simulink library "dspinverses"  (Simulink 8.0)
settings: Solver=ode45  SolverMode=SingleTasking  StartTime=0.0  StopTime=10.0  RelTol=1e-3
libraries: dspmtrx3 x3, dspsolvers x3
settings Model: Creator=dlinebar  LastModifiedBy=lij  ExtModeAutoUpdateStatusClock=off

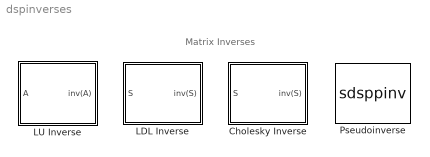
== system dspinverses ==
  note: Matrix Inverses
  " LU Inverse" : Subsystem
      mask Type: LU Inverse
      mask Description: Matrix inverse using LU factorization.
      mask Help: eval('blocksethelp');
      mask Display:
      | text(0.25,0.85,'General')
      | text(0.25,0.70,'Inverse')
      | text(0.35,0.25,'(LU)')
  Cholesky Inverse : Subsystem  mask(Cholesky Inverse){errmode=Warning}
      mask prompts: errmode "Non-positive definite input:"
      mask help: Matrix inverse using Cholesky factorization.
      mask init:
      | set_param([gcb '/Cholesky Solver'],'MaskTunableValues',{'off'});
      | set_param([gcb '/Cholesky Solver'],'errmode',get_param(gcb,'errmode'));
      mask Help: eval('blocksethelp');
      mask StyleString: popup(Ignore|Warning|Error)
      mask Display:
      | text(0.05,0.85,'Sym. Pos. Def.')
      | text(0.25,0.70,'Inverse')
      | text(0.35,0.25,'(Chol)')
  LDL Inverse : Subsystem  mask(LDL Inverse){errmode=Warning}
      mask prompts: errmode "Non-positive definite input:"
      mask help: Matrix inverse using LDL factorization.
      mask init:
      | %
      | set_param([gcb '/LDL Solver'],'errmode',get_param(gcb,'errmode'));
      mask Help: eval('blocksethelp');
      mask StyleString: popup(Ignore|Warning|Error)
      mask Display:
      | text(0.05,0.85,'Sym. Pos. Def.')
      | text(0.25,0.70,'Inverse')
      | text(0.35,0.25,'(LDL)')
  Pseudoinverse : S-Function  FunctionName=sdsppinv  Parameters=wanterr  EnableBusSupport=off  mask(Pseudoinverse){wanterr=off}
      mask prompts: wanterr "Show error status port (E)"
      mask help:
      | X is the Moore-Penrose Pseudoinverse and satisfies 4 criteria: X*A*X=X, A*X*A=A, and A*X and X*A are Hermitian.
      |
      | Select the 'Show error status port (E)' check box to send the SVD convergence error status to an output port.
      mask init:
      | s = dspblkpinv;
      | 
      | % put the following lines in the icon drawing commands box
      | % to get port labels (A on input, A+ on output)
      | 
      | % port_label('input',s.i1,s.i1s);
      | % port_label('output',s.o1,s.o1s);
      mask Help: eval('blocksethelp');
      mask Display:
      | text(0.07,0.75,'Pseudoinverse')
      | text(0.35,0.25,'(SVD)')
      | 
      | port_label('input',s.i1,s.i1s);
      | port_label('output',s.o1,s.o1s);
      | port_label('output',s.o2,s.o2s);

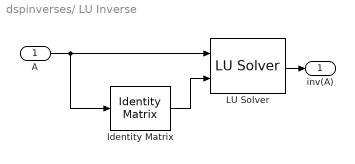
== system dspinverses/ LU Inverse ==
  A : Inport
  Identity Matrix : dspmtrx3/Identity Matrix  Inherit=on  N=5  Ts=1  dataType=double  wordLen=16  udDataType=sfix(16)  fracBitsMode=Best precision  numFracBits=15
  LU Solver : dspsolvers/LU Solver
  inv(A) : Outport
  wires:
  LU Solver/1 -> inv(A)/1
  A/1 -> Identity Matrix/1, LU Solver/1
  Identity Matrix/1 -> LU Solver/2

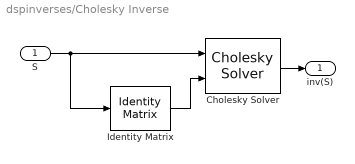
== system dspinverses/Cholesky Inverse ==
  S : Inport
  Cholesky Solver : dspsolvers/Cholesky Solver  errmode=Warning
  Identity Matrix : dspmtrx3/Identity Matrix  Inherit=on  N=5  Ts=1  dataType=double  wordLen=16  udDataType=sfix(16)  fracBitsMode=Best precision  numFracBits=15
  inv(S) : Outport
  wires:
  Cholesky Solver/1 -> inv(S)/1
  S/1 -> Identity Matrix/1, Cholesky Solver/1
  Identity Matrix/1 -> Cholesky Solver/2

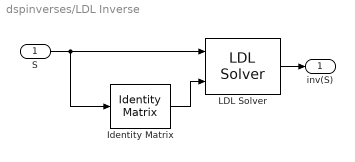
== system dspinverses/LDL Inverse ==
  S : Inport
  Identity Matrix : dspmtrx3/Identity Matrix  Inherit=on  N=5  Ts=1  dataType=double  wordLen=16  udDataType=sfix(16)  fracBitsMode=Best precision  numFracBits=15
  LDL Solver : dspsolvers/LDL Solver  errmode=Warning
  inv(S) : Outport
  wires:
  Identity Matrix/1 -> LDL Solver/2
  S/1 -> LDL Solver/1, Identity Matrix/1
  LDL Solver/1 -> inv(S)/1
